simulink model "myFuzzy"  (R2021a)
settings: Solver=FixedStepAuto  StartTime=0.0  StopTime=inf  FixedStep=0.1  RelTol=1e-3
libraries: robotlib x4, fuzblock x1
settings Model: Creator=bilal  LastModifiedBy=bilal

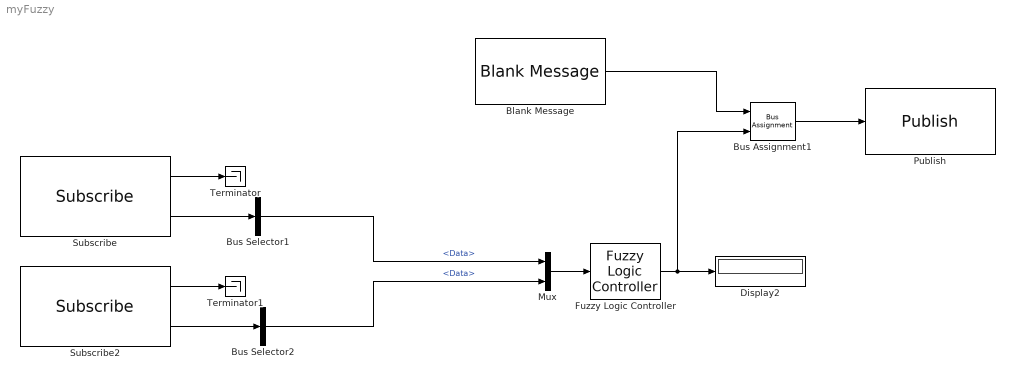
== system myFuzzy ==
  Blank Message : robotlib/Blank Message  messageClass=Message  entityType=std_msgs/Float64  messageType=std_msgs/Float64  SampleTime=inf  legacyBusStruct=off
  Bus Assignment1 : BusAssignment  AssignedSignals=Data
  Bus Selector1 : BusSelector  DialogController=Simulink.DDGSource_BusSelector  OutputSignals=Data
  Bus Selector2 : BusSelector  DialogController=Simulink.DDGSource_BusSelector  OutputSignals=Data
  Display2 : Display
  Fuzzy Logic Controller : fuzblock/Fuzzy Logic  Controller  FIS='R_calculator2.fis'  OutputSampleNumber=101  DataType=double  FuzzifiedInputs=off  RuleFiringStrengths=off  RuleOutputs=off  AggregatedOutputs=off  SimulateUsing=Interpreted execution  OutOfRangeInputValueMessage=warning  NoRuleFiredMessage=warning  EmptyOutputFuzzySetMessage=warning
  Mux : Mux  Inputs=2
  Publish : robotlib/Publish  topicSource=Specify your own  topic=/consider  messageType=std_msgs/Float64  legacyBusStruct=off  messageQueueLength=10
  Subscribe : robotlib/Subscribe  topicSource=Specify your own  topic=/distance  messageType=std_msgs/Float32  SampleTime=-1  legacyBusStruct=off  messageQueueLength=1
  Subscribe2 : robotlib/Subscribe  topicSource=Specify your own  topic=/theta_angle  messageType=std_msgs/Float32  SampleTime=-1  legacyBusStruct=off  messageQueueLength=1
  Terminator : Terminator
  Terminator1 : Terminator
  wires:
  Subscribe/1 -> Terminator/1
  Subscribe2/1 -> Terminator1/1
  Subscribe/2 -> Bus Selector1/1
  Bus Selector1/1 -> Mux/1  "<Data>"
  Subscribe2/2 -> Bus Selector2/1
  Bus Selector2/1 -> Mux/2  "<Data>"
  Mux/1 -> Fuzzy Logic Controller/1
  Bus Assignment1/1 -> Publish/1
  Blank Message/1 -> Bus Assignment1/1
  Fuzzy Logic Controller/1 -> Bus Assignment1/2, Display2/1
